simulink model "NOx_INTEGRATED_GUIDLINE_MODEL"  (R2019a)
settings: Solver=FixedStepDiscrete  StartTime=0.0  StopTime=100  FixedStep=0.1  RelTol=1e-3
values from neighbouring files (symbols this model uses):
  ADblue_CONC_MAX = 34.0    [Integrated_Model_DD.sldd]    (also in NOx_INTEGRATED_PARAMETER_SCRIPT.m = Simulink.Parameter)
  ADblue_CONC_MIN = 33.0    [Integrated_Model_DD.sldd]    (also in NOx_INTEGRATED_PARAMETER_SCRIPT.m = Simulink.Parameter)
  ADblue_LEVEL_MAX = 30.0    [Integrated_Model_DD.sldd]    (also in NOx_INTEGRATED_PARAMETER_SCRIPT.m = Simulink.Parameter)
  ADblue_LEVEL_MIN = 15.0    [Integrated_Model_DD.sldd]    (also in NOx_INTEGRATED_PARAMETER_SCRIPT.m = Simulink.Parameter)
  FLOW_RATE_MIN = 4.8    [Integrated_Model_DD.sldd]    (also in NOx_INTEGRATED_PARAMETER_SCRIPT.m = Simulink.Parameter)
  HEATER = 5.0    [Integrated_Model_DD.sldd]    (also in NOx_INTEGRATED_PARAMETER_SCRIPT.m = Simulink.Parameter)
  NOX_DOWN = 10.0    [Integrated_Model_DD.sldd]    (also in NOx_INTEGRATED_PARAMETER_SCRIPT.m = Simulink.Parameter)
  O2_concentration_max = 14.0    [Integrated_Model_DD.sldd]    (also in NOx_INTEGRATED_PARAMETER_SCRIPT.m = Simulink.Parameter)
  O2_concentration_min = 8.0    [Integrated_Model_DD.sldd]    (also in NOx_INTEGRATED_PARAMETER_SCRIPT.m = Simulink.Parameter)
  PRESSURE_REQ = 5.8    [Integrated_Model_DD.sldd]    (also in NOx_INTEGRATED_PARAMETER_SCRIPT.m = Simulink.Parameter)
  REG_TIME_OFF = 25.0    [Integrated_Model_DD.sldd]    (also in NOx_INTEGRATED_PARAMETER_SCRIPT.m = Simulink.Parameter)
  SCR_BED_TEMP_MIN = 200.0    [Integrated_Model_DD.sldd]    (also in NOx_INTEGRATED_PARAMETER_SCRIPT.m = Simulink.Parameter)
  soot_max = 0.45    [Integrated_Model_DD.sldd]    (also in NOx_INTEGRATED_PARAMETER_SCRIPT.m = Simulink.Parameter)
  soot_mil = 0.9    [Integrated_Model_DD.sldd]    (also in NOx_INTEGRATED_PARAMETER_SCRIPT.m = Simulink.Parameter)
  Time_off = 0.0    [Integrated_Model_DD.sldd]    (also in NOx_INTEGRATED_PARAMETER_SCRIPT.m = Simulink.Parameter)
  Time_on = 1.0    [Integrated_Model_DD.sldd]    (also in NOx_INTEGRATED_PARAMETER_SCRIPT.m = Simulink.Parameter)
  TIMER = 0.1    [Integrated_Model_DD.sldd]    (also in NOx_INTEGRATED_PARAMETER_SCRIPT.m = Simulink.Parameter)
settings Model: Creator=User  LastModifiedBy=User
settings OptimizationCC: DefaultParameterBehavior=Inlined  EnhancedBackFolding=on  PassReuseOutputArgsAs=Individual arguments  OptimizeBlockOrder=speed  DifferentSizesBufferReuse=on  OptimizationCustomize=off
settings DebuggingCC: SignalInfNanChecking=warning  ParameterTunabilityLossMsg=error  UniqueDataStoreMsg=warning  StrictBusMsg=ErrorOnBusTreatedAsVector
settings SFSimCC: MATLABDynamicMemAlloc=off
settings RTWCC: SystemTargetFile=ert.tlc  GenCodeOnly=on  TemplateMakefile=ert_default_tmf  GenerateReport=on  IncludeHyperlinkInReport=on  LaunchReport=on  GenerateTraceInfo=on  GenerateTraceReport=on  GenerateTraceReportSl=on  GenerateTraceReportSf=on  GenerateTraceReportEml=on
settings CodeAppCC: ForceParamTrailComments=on  IgnoreCustomStorageClasses=off  OperatorAnnotations=on  SimulinkDataObjDesc=on  SFDataObjDesc=on  InsertBlockDesc=on
settings ERTTargetCC: TargetLangStandard=C99 (ISO)  GenerateSampleERTMain=on  InlinedParameterPlacement=NonHierarchical  ERTCustomFileTemplate=example_file_process.tlc

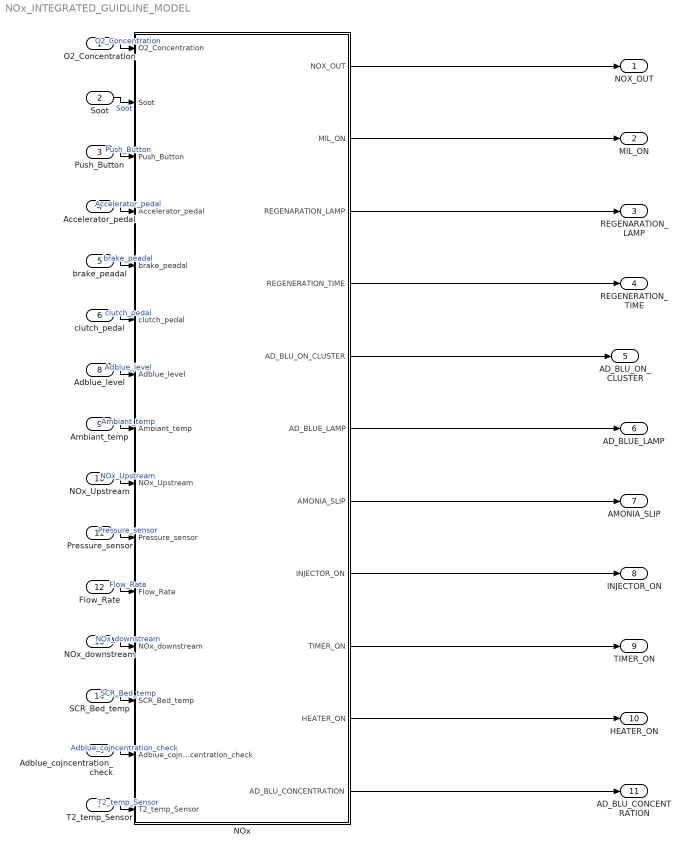
== system NOx_INTEGRATED_GUIDLINE_MODEL ==
  O2_Concentration : Inport
  Soot : Inport  Port=2
  Push_Button : Inport  Port=3
  Accelerator_pedal : Inport  Port=4
  brake_peadal : Inport  Port=5
  clutch_pedal : Inport  Port=6
  T2_temp_Sensor : Inport  Port=7
  Adblue_level : Inport  Port=8
  Ambiant_temp : Inport  Port=9
  NOx_Upstream : Inport  Port=10
  Pressure_sensor : Inport  Port=11
  Flow_Rate : Inport  Port=12
  NOx_downstream : Inport  Port=13
  SCR_Bed_temp : Inport  Port=14
  Adblue_cojncentration_check : Inport  Port=15
  NOx : Subsystem  TreatAsAtomicUnit=on
  NOX_OUT : Outport
  MIL_ON : Outport  Port=2
  REGENARATION_LAMP : Outport  Port=3
  REGENERATION_TIME : Outport  Port=4
  AD_BLU_ON_CLUSTER : Outport  Port=5
  AD_BLUE_LAMP : Outport  Port=6
  AMONIA_SLIP : Outport  Port=7
  INJECTOR_ON : Outport  Port=8
  TIMER_ON : Outport  Port=9
  HEATER_ON : Outport  Port=10
  AD_BLU_CONCENTRATION : Outport  Port=11
  wires:
  Adblue_cojncentration_check/1 -> NOx/14(Adblue_cojncentration_check)  "Adblue_cojncentration_check"
  Pressure_sensor/1 -> NOx/10(Pressure_sensor)  "Pressure_sensor"
  Flow_Rate/1 -> NOx/11(Flow_Rate)  "Flow_Rate"
  T2_temp_Sensor/1 -> NOx/15(T2_temp_Sensor)  "T2_temp_Sensor"
  SCR_Bed_temp/1 -> NOx/13(SCR_Bed_temp)  "SCR_Bed_temp"
  Soot/1 -> NOx/2(Soot)  "Soot"
  NOx_downstream/1 -> NOx/12(NOx_downstream)  "NOx_downstream"
  NOx_Upstream/1 -> NOx/9(NOx_Upstream)  "NOx_Upstream"
  O2_Concentration/1 -> NOx/1(O2_Concentration)  "O2_Concentration"
  Ambiant_temp/1 -> NOx/8(Ambiant_temp)  "Ambiant_temp"
  brake_peadal/1 -> NOx/5(brake_peadal)  "brake_peadal"
  Accelerator_pedal/1 -> NOx/4(Accelerator_pedal)  "Accelerator_pedal"
  Push_Button/1 -> NOx/3(Push_Button)  "Push_Button"
  clutch_pedal/1 -> NOx/6(clutch_pedal)  "clutch_pedal"
  Adblue_level/1 -> NOx/7(Adblue_level)  "Adblue_level"
  NOx/2(MIL_ON) -> MIL_ON/1
  NOx/11(AD_BLU_CONCENTRATION) -> AD_BLU_CONCENTRATION/1
  NOx/6(AD_BLUE_LAMP) -> AD_BLUE_LAMP/1
  NOx/1(NOX_OUT) -> NOX_OUT/1
  NOx/7(AMONIA_SLIP) -> AMONIA_SLIP/1
  NOx/4(REGENERATION_TIME) -> REGENERATION_TIME/1
  NOx/3(REGENARATION_LAMP) -> REGENARATION_LAMP/1
  NOx/8(INJECTOR_ON) -> INJECTOR_ON/1
  NOx/5(AD_BLU_ON_CLUSTER) -> AD_BLU_ON_CLUSTER/1
  NOx/10(HEATER_ON) -> HEATER_ON/1
  NOx/9(TIMER_ON) -> TIMER_ON/1

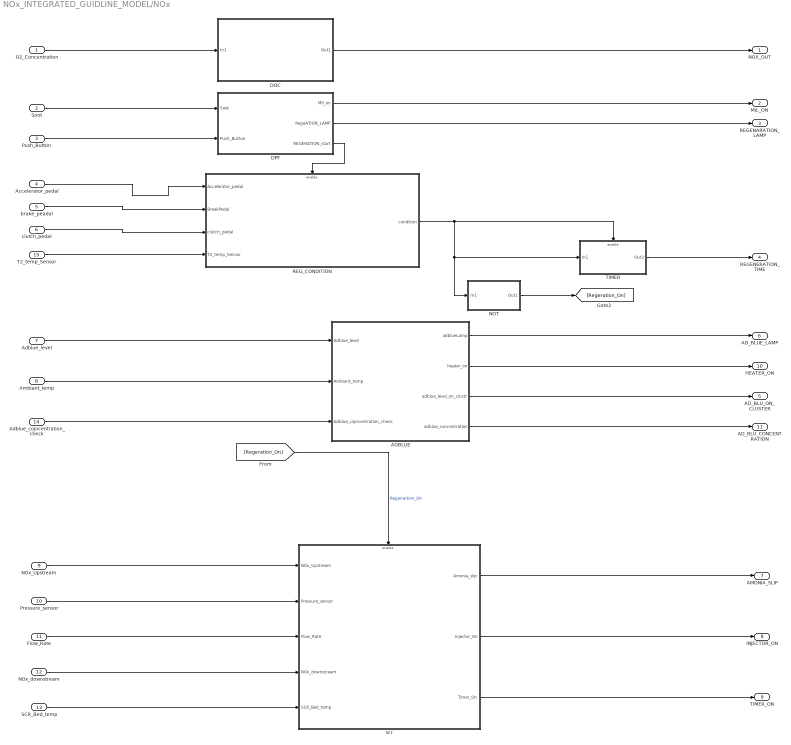
== system NOx_INTEGRATED_GUIDLINE_MODEL/NOx ==
  O2_Concentration : Inport
  Soot : Inport  Port=2
  Push_Button : Inport  Port=3
  Accelerator_pedal : Inport  Port=4
  brake_peadal : Inport  Port=5
  clutch_pedal : Inport  Port=6
  Adblue_level : Inport  Port=7
  Ambiant_temp : Inport  Port=8
  NOx_Upstream : Inport  Port=9
  Pressure_sensor : Inport  Port=10
  Flow_Rate : Inport  Port=11
  NOx_downstream : Inport  Port=12
  SCR_Bed_temp : Inport  Port=13
  Adblue_cojncentration_check : Inport  Port=14
  T2_temp_Sensor : Inport  Port=15
  ADBLUE : Subsystem  TreatAsAtomicUnit=on
  DOC : Subsystem  TreatAsAtomicUnit=on
  DPF : Subsystem  TreatAsAtomicUnit=on
  NOT : Subsystem  TreatAsAtomicUnit=on
  REG_CONDITION : Subsystem
  TIMER : Subsystem
  scr : Subsystem
  NOX_OUT : Outport
  MIL_ON : Outport  Port=2
  REGENARATION_LAMP : Outport  Port=3
  REGENERATION_TIME : Outport  Port=4
  AD_BLU_ON_CLUSTER : Outport  Port=5
  AD_BLUE_LAMP : Outport  Port=6
  AMONIA_SLIP : Outport  Port=7
  INJECTOR_ON : Outport  Port=8
  TIMER_ON : Outport  Port=9
  HEATER_ON : Outport  Port=10
  AD_BLU_CONCENTRATION : Outport  Port=11
  wires:
  scr/3(Timer_On) -> TIMER_ON/1
  Push_Button/1 -> DPF/2(Push_Button)
  DPF/3(REGERATION_start) -> REG_CONDITION/Enable
  scr/1(Amonia_slip) -> AMONIA_SLIP/1
  NOx_Upstream/1 -> scr/1(NOx_Upstream)
  DOC/1(Out1) -> NOX_OUT/1
  DPF/2(RegeATION_LAMP) -> REGENARATION_LAMP/1
  [Regeration_On] -> scr/Enable  "Regenartion_On"
  Adblue_level/1 -> ADBLUE/1(Adblue_level)
  O2_Concentration/1 -> DOC/1(In1)
  Accelerator_pedal/1 -> REG_CONDITION/1(Accelerator_pedal)
  Flow_Rate/1 -> scr/3(Flow_Rate)
  Soot/1 -> DPF/1(Soot)
  Pressure_sensor/1 -> scr/2(Pressure_sensor)
  scr/2(Injector_On) -> INJECTOR_ON/1
  NOx_downstream/1 -> scr/4(NOx_downstream)
  SCR_Bed_temp/1 -> scr/5(SCR_Bed_temp)
  DPF/1(MIl_on) -> MIL_ON/1
  Ambiant_temp/1 -> ADBLUE/2(Ambiant_temp)
  ADBLUE/1(adblueLamp) -> AD_BLUE_LAMP/1
  ADBLUE/3(adblue_level_on_clustr) -> AD_BLU_ON_CLUSTER/1
  ADBLUE/2(heater_on) -> HEATER_ON/1
  Adblue_cojncentration_check/1 -> ADBLUE/3(Adblue_cojncentration_check)
  ADBLUE/4(adblue_concentration) -> AD_BLU_CONCENTRATION/1
  TIMER/1(Out2) -> REGENERATION_TIME/1
  clutch_pedal/1 -> REG_CONDITION/3(clutch_pedal)
  brake_peadal/1 -> REG_CONDITION/2(BreakPedal)
  T2_temp_Sensor/1 -> REG_CONDITION/4(T2_temp_Sensor)
  NOT/1(Out1) -> [Regeration_On]
  REG_CONDITION/1(condition) -> TIMER/1(In1), NOT/1(In1), TIMER/Enable

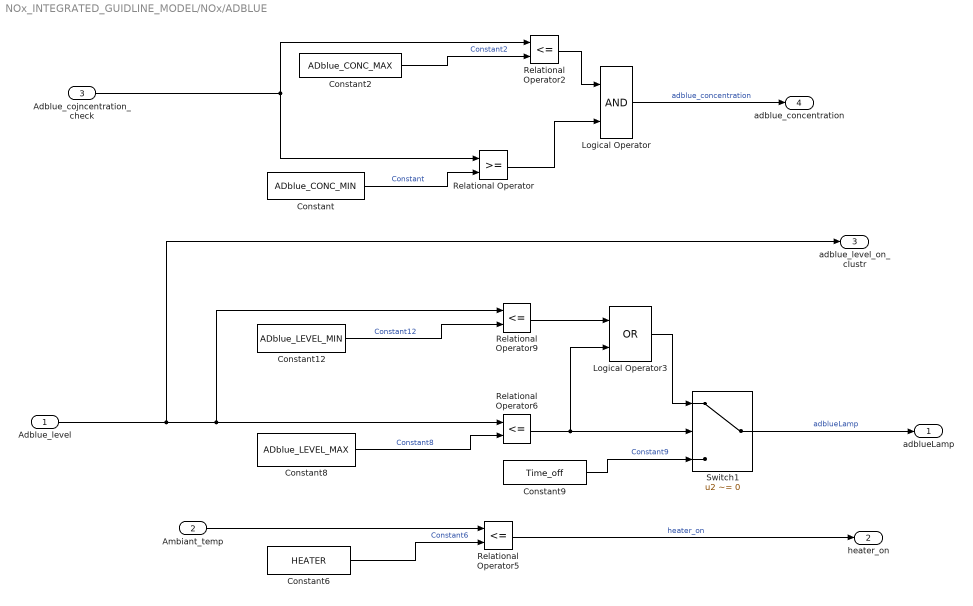
== system NOx_INTEGRATED_GUIDLINE_MODEL/NOx/ADBLUE ==
  Adblue_level : Inport
  Ambiant_temp : Inport  Port=2
  Adblue_cojncentration_check : Inport  Port=3
  Constant : Constant  Value=ADblue_CONC_MIN
  Constant12 : Constant  Value=ADblue_LEVEL_MIN
  Constant2 : Constant  Value=ADblue_CONC_MAX
  Constant6 : Constant  Value=HEATER  OutDataTypeStr=int8
  Constant8 : Constant  Value=ADblue_LEVEL_MAX
  Constant9 : Constant  Value=Time_off
  Logical Operator : Logic  AllPortsSameDT=off  OutDataTypeStr=boolean
  Logical Operator3 : Logic  Operator=OR  AllPortsSameDT=off  OutDataTypeStr=boolean
  Relational Operator : RelationalOperator  OutDataTypeStr=boolean  RndMeth=Simplest
  Relational Operator{2,5..6,9} (4 alike) : RelationalOperator  Operator=<=  OutDataTypeStr=boolean  RndMeth=Simplest
  Switch1 : Switch  Criteria=u2 ~= 0
  adblueLamp : Outport
  heater_on : Outport  Port=2
  adblue_level_on_clustr : Outport  Port=3
  adblue_concentration : Outport  Port=4
  wires:
  Logical Operator3/1 -> Switch1/1
  Constant9/1 -> Switch1/3  "Constant9"
  Adblue_level/1 -> adblue_level_on_clustr/1, Relational Operator6/1, Relational Operator9/1
  Constant8/1 -> Relational Operator6/2  "Constant8"
  Constant12/1 -> Relational Operator9/2  "Constant12"
  Relational Operator6/1 -> Logical Operator3/2, Switch1/2
  Constant6/1 -> Relational Operator5/2  "Constant6"
  Relational Operator5/1 -> heater_on/1  "heater_on"
  Switch1/1 -> adblueLamp/1  "adblueLamp"
  Ambiant_temp/1 -> Relational Operator5/1
  Constant/1 -> Relational Operator/2  "Constant"
  Constant2/1 -> Relational Operator2/2  "Constant2"
  Relational Operator2/1 -> Logical Operator/1
  Adblue_cojncentration_check/1 -> Relational Operator/1, Relational Operator2/1
  Logical Operator/1 -> adblue_concentration/1  "adblue_concentration"
  Relational Operator/1 -> Logical Operator/2
  Relational Operator9/1 -> Logical Operator3/1

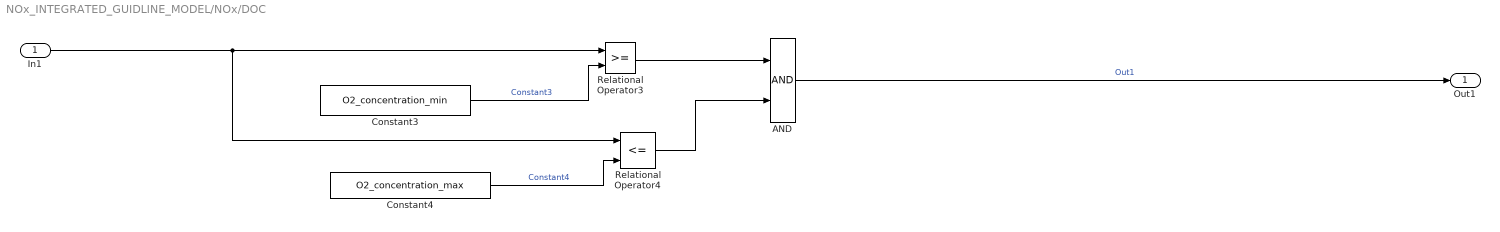
== system NOx_INTEGRATED_GUIDLINE_MODEL/NOx/DOC ==
  In1 : Inport
  AND : Logic  AllPortsSameDT=off  OutDataTypeStr=boolean
  Constant3 : Constant  Value=O2_concentration_min
  Constant4 : Constant  Value=O2_concentration_max
  Relational Operator3 : RelationalOperator  OutDataTypeStr=boolean  RndMeth=Simplest
  Relational Operator4 : RelationalOperator  Operator=<=  OutDataTypeStr=boolean  RndMeth=Simplest
  Out1 : Outport
  wires:
  Constant3/1 -> Relational Operator3/2  "Constant3"
  Relational Operator3/1 -> AND/1
  AND/1 -> Out1/1  "Out1"
  In1/1 -> Relational Operator4/1, Relational Operator3/1
  Constant4/1 -> Relational Operator4/2  "Constant4"
  Relational Operator4/1 -> AND/2

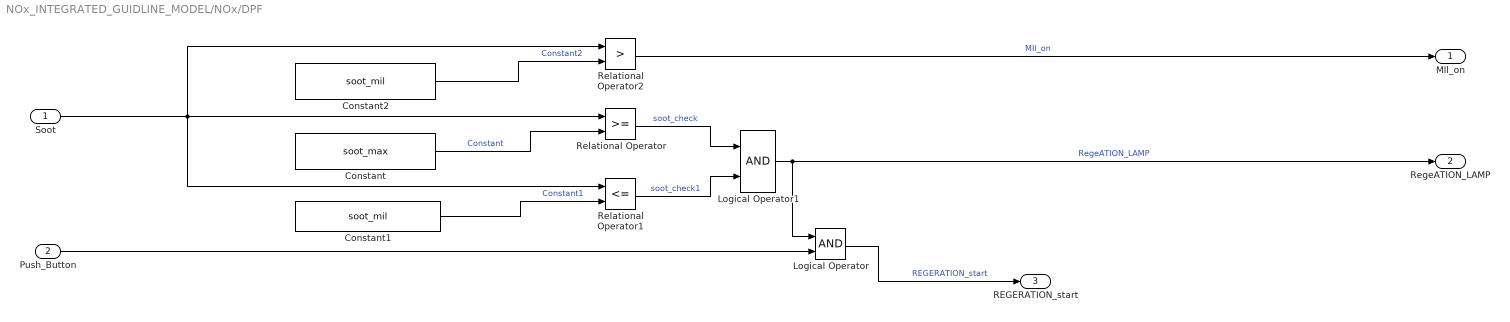
== system NOx_INTEGRATED_GUIDLINE_MODEL/NOx/DPF ==
  Soot : Inport
  Push_Button : Inport  Port=2
  Constant : Constant  Value=soot_max
  Constant1 : Constant  Value=soot_mil
  Constant2 : Constant  Value=soot_mil
  Logical Operator : Logic  AllPortsSameDT=off  OutDataTypeStr=boolean
  Logical Operator1 : Logic  AllPortsSameDT=off  OutDataTypeStr=boolean
  Relational Operator : RelationalOperator  OutDataTypeStr=boolean  RndMeth=Simplest
  Relational Operator1 : RelationalOperator  Operator=<=  OutDataTypeStr=boolean  RndMeth=Simplest
  Relational Operator2 : RelationalOperator  Operator=>  OutDataTypeStr=boolean  RndMeth=Simplest
  MIl_on : Outport
  RegeATION_LAMP : Outport  Port=2
  REGERATION_start : Outport  Port=3
  wires:
  Soot/1 -> Relational Operator1/1, Relational Operator2/1, Relational Operator/1
  Logical Operator/1 -> REGERATION_start/1  "REGERATION_start"
  Logical Operator1/1 -> RegeATION_LAMP/1, Logical Operator/1  "RegeATION_LAMP"
  Constant2/1 -> Relational Operator2/2  "Constant2"
  Push_Button/1 -> Logical Operator/2
  Constant1/1 -> Relational Operator1/2  "Constant1"
  Constant/1 -> Relational Operator/2  "Constant"
  Relational Operator1/1 -> Logical Operator1/2  "soot_check1"
  Relational Operator2/1 -> MIl_on/1  "MIl_on"
  Relational Operator/1 -> Logical Operator1/1  "soot_check"

== system NOx_INTEGRATED_GUIDLINE_MODEL/NOx/NOT ==
  In1 : Inport
  NOT : Logic  Operator=NOT  IconShape=distinctive  AllPortsSameDT=off  OutDataTypeStr=boolean
  Out1 : Outport
  wires:
  In1/1 -> NOT/1
  NOT/1 -> Out1/1  "not_out"

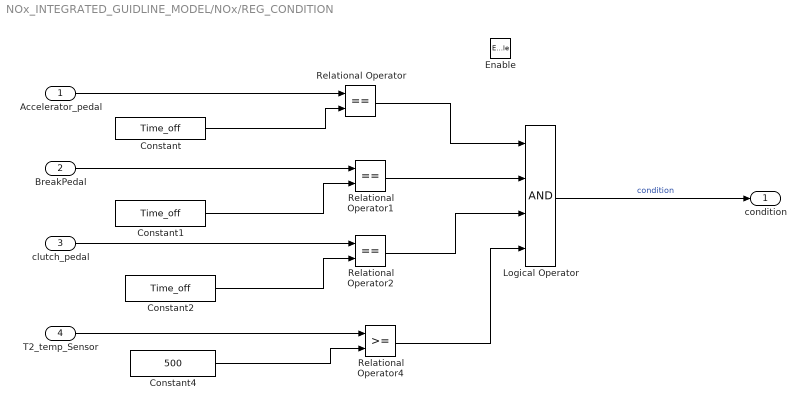
== system NOx_INTEGRATED_GUIDLINE_MODEL/NOx/REG_CONDITION ==
  Accelerator_pedal : Inport
  BreakPedal : Inport  Port=2
  clutch_pedal : Inport  Port=3
  T2_temp_Sensor : Inport  Port=4
  Enable : EnablePort  StatesWhenEnabling=reset
  Constant : Constant  Value=Time_off
  Constant1 : Constant  Value=Time_off
  Constant2 : Constant  Value=Time_off
  Constant4 : Constant  Value=500
  Logical Operator : Logic  Inputs=4  AllPortsSameDT=off
  Relational Operator : RelationalOperator  Operator===  OutDataTypeStr=boolean  RndMeth=Simplest
  Relational Operator1 : RelationalOperator  Operator===  OutDataTypeStr=boolean  RndMeth=Simplest
  Relational Operator2 : RelationalOperator  Operator===  OutDataTypeStr=boolean  RndMeth=Simplest
  Relational Operator4 : RelationalOperator  OutDataTypeStr=boolean  RndMeth=Simplest
  condition : Outport
  wires:
  Constant/1 -> Relational Operator/2
  Accelerator_pedal/1 -> Relational Operator/1
  Constant1/1 -> Relational Operator1/2
  Constant2/1 -> Relational Operator2/2
  Relational Operator/1 -> Logical Operator/1
  Relational Operator1/1 -> Logical Operator/2
  Relational Operator2/1 -> Logical Operator/3
  Constant4/1 -> Relational Operator4/2
  Logical Operator/1 -> condition/1  "condition"
  Relational Operator4/1 -> Logical Operator/4
  BreakPedal/1 -> Relational Operator1/1
  clutch_pedal/1 -> Relational Operator2/1
  T2_temp_Sensor/1 -> Relational Operator4/1

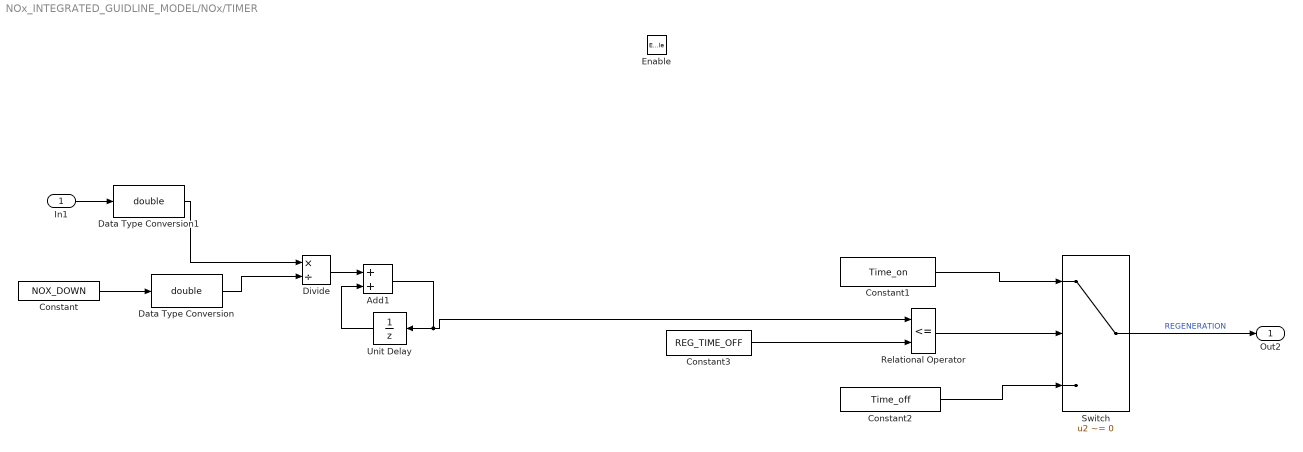
== system NOx_INTEGRATED_GUIDLINE_MODEL/NOx/TIMER ==
  In1 : Inport
  Enable : EnablePort  StatesWhenEnabling=reset
  Add1 : Sum  OutDataTypeStr=double
  Constant : Constant  Value=NOX_DOWN  OutDataTypeStr=double
  Constant1 : Constant  Value=Time_on
  Constant2 : Constant  Value=Time_off
  Constant3 : Constant  Value=REG_TIME_OFF
  Data Type Conversion : DataTypeConversion  OutDataTypeStr=double
  Data Type Conversion1 : DataTypeConversion  OutDataTypeStr=double
  Divide : Product  Inputs=*/  OutDataTypeStr=double
  Relational Operator : RelationalOperator  Operator=<=  OutDataTypeStr=boolean  RndMeth=Simplest
  Switch : Switch  Criteria=u2 ~= 0
  Unit Delay : UnitDelay  InitialCondition=0.1  SampleTime=-1  HasFrameUpgradeWarning=on
  Out2 : Outport
  wires:
  Unit Delay/1 -> Add1/2
  Divide/1 -> Add1/1
  Constant/1 -> Data Type Conversion/1
  Add1/1 -> Relational Operator/1, Unit Delay/1
  Constant2/1 -> Switch/3
  Constant3/1 -> Relational Operator/2
  Switch/1 -> Out2/1  "REGENERATION"
  Relational Operator/1 -> Switch/2
  Constant1/1 -> Switch/1
  In1/1 -> Data Type Conversion1/1
  Data Type Conversion/1 -> Divide/2
  Data Type Conversion1/1 -> Divide/1

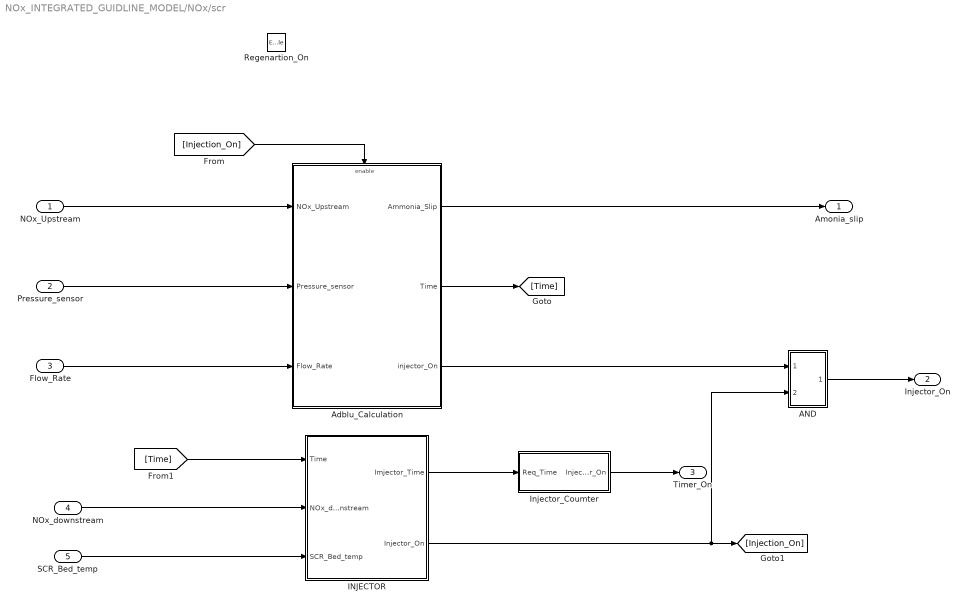
== system NOx_INTEGRATED_GUIDLINE_MODEL/NOx/scr ==
  NOx_Upstream : Inport
  Pressure_sensor : Inport  Port=2
  Flow_Rate : Inport  Port=3
  NOx_downstream : Inport  Port=4
  SCR_Bed_temp : Inport  Port=5
  Regenartion_On : EnablePort
  AND : Subsystem  TreatAsAtomicUnit=on
  Adblu_Calculation : Subsystem
  INJECTOR : Subsystem
  Injector_Coumter : Subsystem  TreatAsAtomicUnit=on
  Amonia_slip : Outport
  Injector_On : Outport  Port=2
  Timer_On : Outport  Port=3
  wires:
  Adblu_Calculation/2(Time) -> [Time]
  [Time] -> INJECTOR/1(Time)
  Injector_Coumter/1(Injector_On) -> Timer_On/1
  INJECTOR/2(Injector_On) -> [Injection_On], AND/2(In2)
  INJECTOR/1(Imjector_Time) -> Injector_Coumter/1(Req_Time)
  [Injection_On] -> Adblu_Calculation/Enable
  Adblu_Calculation/1(Ammonia_Slip) -> Amonia_slip/1
  NOx_downstream/1 -> INJECTOR/2(NOx_downstream)
  NOx_Upstream/1 -> Adblu_Calculation/1(NOx_Upstream)
  SCR_Bed_temp/1 -> INJECTOR/3(SCR_Bed_temp)
  Pressure_sensor/1 -> Adblu_Calculation/2(Pressure_sensor)
  Flow_Rate/1 -> Adblu_Calculation/3(Flow_Rate)
  Adblu_Calculation/3(injector_On) -> AND/1(In1)
  AND/1(Out1) -> Injector_On/1

== system NOx_INTEGRATED_GUIDLINE_MODEL/NOx/scr/AND ==
  In1 : Inport
  In2 : Inport  Port=2
  Logical Operator2 : Logic  AllPortsSameDT=off  OutDataTypeStr=boolean
  Out1 : Outport
  wires:
  In2/1 -> Logical Operator2/2
  Logical Operator2/1 -> Out1/1  "Out1"
  In1/1 -> Logical Operator2/1

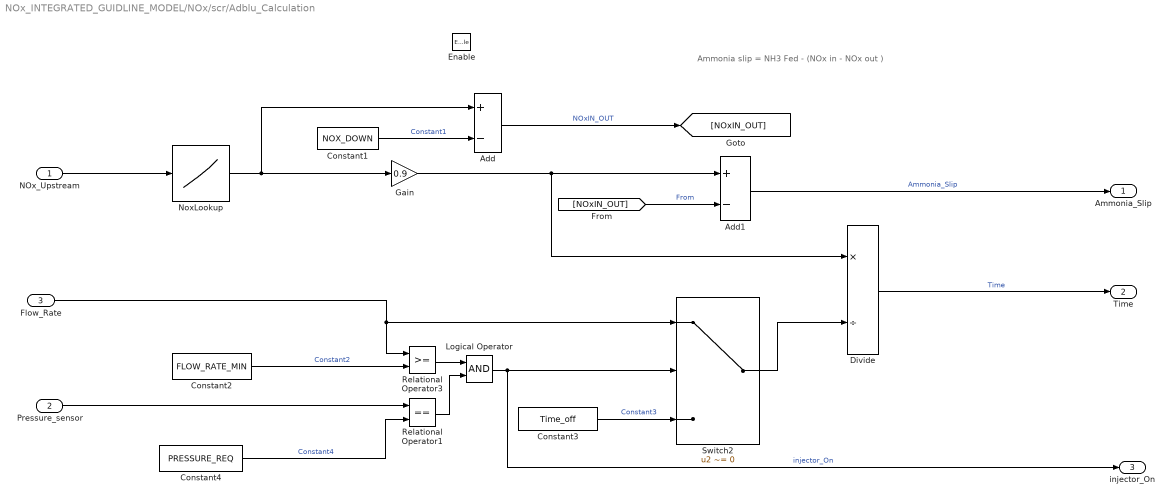
== system NOx_INTEGRATED_GUIDLINE_MODEL/NOx/scr/Adblu_Calculation ==
  note: Ammonia slip = NH3 Fed - (NOx in - NOx out )
  NOx_Upstream : Inport
  Pressure_sensor : Inport  Port=2
  Flow_Rate : Inport  Port=3
  Enable : EnablePort  StatesWhenEnabling=reset
  Add : Sum  Inputs=+-
  Add1 : Sum  Inputs=+-
  Constant1 : Constant  Value=NOX_DOWN
  Constant2 : Constant  Value=FLOW_RATE_MIN
  Constant3 : Constant  Value=Time_off
  Constant4 : Constant  Value=PRESSURE_REQ
  Divide : Product  Inputs=*/  OutDataTypeStr=double  RndMeth=Round
  Gain : Gain  Gain=0.9
  Logical Operator : Logic  AllPortsSameDT=off  OutDataTypeStr=boolean
  NoxLookup : Lookup_n-D  NumberOfTableDimensions=1  BreakpointsForDimension1=|  BreakpointsForDimension1DataTypeStr=double  Table=|  TableDataTypeStr=double  IntermediateResultsDataTypeStr=double  InternalRulePriority=Speed  OutDataTypeStr=double  InputSameDT=on
      BreakpointsForDimension1=|
      | [10
      | 70
      | 77.6
      | 80.4
      | 86.4
      | 99.6
      | 108
      | 117.6
      | 127.2
      | 136.8
      | 149.3
      | 158.3
      | 163.3
      | 168.3
      | 175.3
      | 181.5
      | 187.7
      | 193.9
      | 200.1
      | 206.3
      | 212.85
      | 223.5
      | 233.15
      | 242.8
      | 255.45
      | 264.9
      | 275.35
      | 285.8
      | 296.25
      | 306.7
      | 317.15
      | 327.6
      | 338.05
      | 348.5
      | 358.95
      | 369.4
      | 379.85
      | 390.3
      | 400.75
      | 411.2
      | 421.65
      | 432.1
      | 442.55
      | 453
      | 463.45
      | 473.9
      | 484.35
      | 494.8
      | 505.25
      | 515.7
      | 526.15
      | 536.6
      | 547.05
      | 557.5
      | 567.95
      | 578.4
      | 588.85
      | 599.3
      | 609.75
      | 620.2
      | 630.65
      | 641.1
      | 651.55
      | 662
      | 672.45
      | 682.9
      | 693.35
      | 703.8
      | ]
      Table=|
      | [10
      | 70
      | 77.6
      | 80.4
      | 86.4
      | 99.6
      | 108
      | 117.6
      | 127.2
      | 136.8
      | 149.3
      | 158.3
      | 163.3
      | 168.3
      | 175.3
      | 181.5
      | 187.7
      | 193.9
      | 200.1
      | 206.3
      | 212.85
      | 223.5
      | 233.15
      | 242.8
      | 255.45
      | 264.9
      | 275.35
      | 285.8
      | 296.25
      | 306.7
      | 317.15
      | 327.6
      | 338.05
      | 348.5
      | 358.95
      | 369.4
      | 379.85
      | 390.3
      | 400.75
      | 411.2
      | 421.65
      | 432.1
      | 442.55
      | 453
      | 463.45
      | 473.9
      | 484.35
      | 494.8
      | 505.25
      | 515.7
      | 526.15
      | 536.6
      | 547.05
      | 557.5
      | 567.95
      | 578.4
      | 588.85
      | 599.3
      | 609.75
      | 620.2
      | 630.65
      | 641.1
      | 651.55
      | 662
      | 672.45
      | 682.9
      | 693.35
      | 703.8
      | ]
  Relational Operator1 : RelationalOperator  Operator===  OutDataTypeStr=boolean  RndMeth=Simplest
  Relational Operator3 : RelationalOperator  OutDataTypeStr=boolean  RndMeth=Simplest
  Switch2 : Switch  Criteria=u2 ~= 0
  Ammonia_Slip : Outport
  Time : Outport  Port=2
  injector_On : Outport  Port=3
  wires:
  Pressure_sensor/1 -> Relational Operator1/1
  Add/1 -> [NOxIN_OUT]  "NOxIN_OUT"
  Constant1/1 -> Add/2  "Constant1"
  Relational Operator1/1 -> Logical Operator/2
  Constant4/1 -> Relational Operator1/2  "Constant4"
  NOx_Upstream/1 -> NoxLookup/1
  Constant2/1 -> Relational Operator3/2  "Constant2"
  Relational Operator3/1 -> Logical Operator/1
  Constant3/1 -> Switch2/3  "Constant3"
  Switch2/1 -> Divide/2
  Logical Operator/1 -> injector_On/1, Switch2/2  "injector_On"
  [NOxIN_OUT] -> Add1/2  "From"
  Flow_Rate/1 -> Relational Operator3/1, Switch2/1
  Add1/1 -> Ammonia_Slip/1  "Ammonia_Slip"
  Gain/1 -> Divide/1, Add1/1
  Divide/1 -> Time/1  "Time"
  NoxLookup/1 -> Gain/1, Add/1

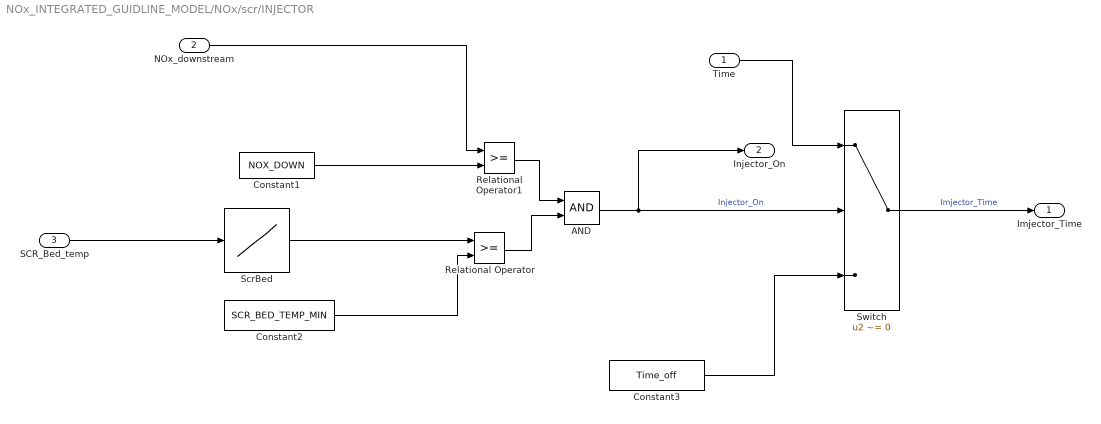
== system NOx_INTEGRATED_GUIDLINE_MODEL/NOx/scr/INJECTOR ==
  Time : Inport
  NOx_downstream : Inport  Port=2
  SCR_Bed_temp : Inport  Port=3
  AND : Logic  AllPortsSameDT=off  OutDataTypeStr=boolean
  Constant1 : Constant  Value=NOX_DOWN
  Constant2 : Constant  Value=SCR_BED_TEMP_MIN
  Constant3 : Constant  Value=Time_off
  Relational Operator : RelationalOperator  OutDataTypeStr=boolean  RndMeth=Simplest
  Relational Operator1 : RelationalOperator  OutDataTypeStr=boolean  RndMeth=Simplest
  ScrBed : Lookup_n-D  NumberOfTableDimensions=1  BreakpointsForDimension1=[1:10:650]  BreakpointsForDimension2=[1:1:500]  BreakpointsForDimension1DataTypeStr=double  Table=[1:10:650]  TableDataTypeStr=double  IntermediateResultsDataTypeStr=double  InternalRulePriority=Speed  OutDataTypeStr=double  InputSameDT=on
  Switch : Switch  Criteria=u2 ~= 0
  Imjector_Time : Outport
  Injector_On : Outport  Port=2
  wires:
  Constant1/1 -> Relational Operator1/2
  Constant2/1 -> Relational Operator/2
  Constant3/1 -> Switch/3
  ScrBed/1 -> Relational Operator/1
  AND/1 -> Injector_On/1, Switch/2  "Injector_On"
  Time/1 -> Switch/1
  Relational Operator1/1 -> AND/1
  Relational Operator/1 -> AND/2
  SCR_Bed_temp/1 -> ScrBed/1
  Switch/1 -> Imjector_Time/1  "Imjector_Time"
  NOx_downstream/1 -> Relational Operator1/1

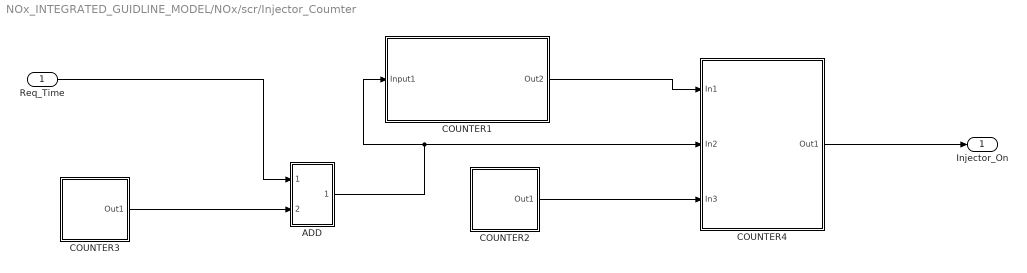
== system NOx_INTEGRATED_GUIDLINE_MODEL/NOx/scr/Injector_Coumter ==
  Req_Time : Inport
  ADD : Subsystem
  COUNTER1 : Subsystem
  COUNTER2 : Subsystem
  COUNTER3 : Subsystem
  COUNTER4 : Subsystem
  Injector_On : Outport
  wires:
  ADD/1(Out1) -> COUNTER4/2(In2), COUNTER1/1(Input1)
  Req_Time/1 -> ADD/1(In1)
  COUNTER1/1(Out2) -> COUNTER4/1(In1)
  COUNTER4/1(Out1) -> Injector_On/1
  COUNTER3/1(Out1) -> ADD/2(In2)
  COUNTER2/1(Out1) -> COUNTER4/3(In3)

== system NOx_INTEGRATED_GUIDLINE_MODEL/NOx/scr/Injector_Coumter/ADD ==
  In1 : Inport
  In2 : Inport  Port=2
  Add1 : Sum
  Relational Operator1 : RelationalOperator  OutDataTypeStr=boolean  RndMeth=Simplest
  Unit Delay : UnitDelay  SampleTime=-1  HasFrameUpgradeWarning=on
  Out1 : Outport
  wires:
  Unit Delay/1 -> Add1/2
  Add1/1 -> Unit Delay/1, Relational Operator1/2
  Relational Operator1/1 -> Out1/1  "Out1"
  In1/1 -> Relational Operator1/1
  In2/1 -> Add1/1

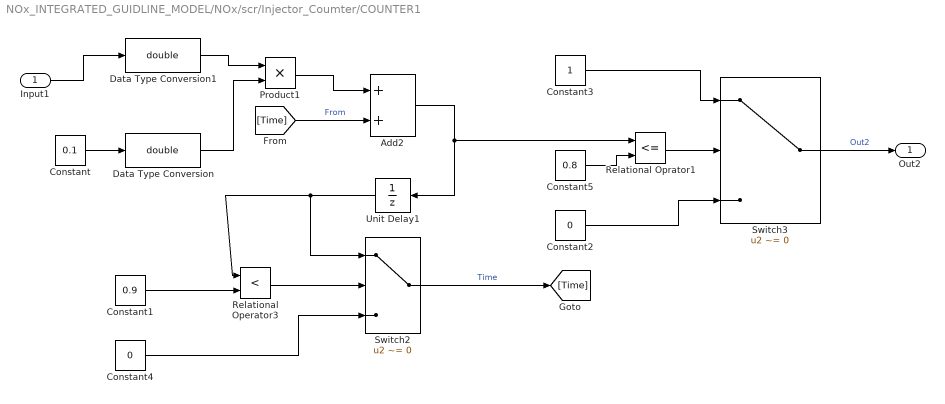
== system NOx_INTEGRATED_GUIDLINE_MODEL/NOx/scr/Injector_Coumter/COUNTER1 ==
  Input1 : Inport
  Add2 : Sum
  Constant : Constant  Value=0.1
  Constant1 : Constant  Value=0.9
  Constant2 : Constant  Value=0
  Constant3 : Constant
  Constant4 : Constant  Value=0
  Constant5 : Constant  Value=0.8
  Data Type Conversion : DataTypeConversion  OutDataTypeStr=double
  Data Type Conversion1 : DataTypeConversion  OutDataTypeStr=double
  Product1 : Product
  Relational Operator3 : RelationalOperator  Operator=<  OutDataTypeStr=boolean  RndMeth=Simplest
  Relational Oprator1 : RelationalOperator  Operator=<=  OutDataTypeStr=boolean  RndMeth=Simplest
  Switch2 : Switch  Criteria=u2 ~= 0
  Switch3 : Switch  Criteria=u2 ~= 0
  Unit Delay1 : UnitDelay  SampleTime=-1  HasFrameUpgradeWarning=on
  Out2 : Outport
  wires:
  Unit Delay1/1 -> Relational Operator3/1, Switch2/1
  Relational Operator3/1 -> Switch2/2
  Constant3/1 -> Switch3/1
  Switch3/1 -> Out2/1  "Out2"
  Constant5/1 -> Relational Oprator1/2
  Constant/1 -> Data Type Conversion/1
  Switch2/1 -> [Time]  "Time"
  Product1/1 -> Add2/1
  Constant1/1 -> Relational Operator3/2
  Constant4/1 -> Switch2/3
  Input1/1 -> Data Type Conversion1/1
  Constant2/1 -> Switch3/3
  [Time] -> Add2/2  "From"
  Relational Oprator1/1 -> Switch3/2
  Add2/1 -> Relational Oprator1/1, Unit Delay1/1
  Data Type Conversion/1 -> Product1/2
  Data Type Conversion1/1 -> Product1/1

== system NOx_INTEGRATED_GUIDLINE_MODEL/NOx/scr/Injector_Coumter/COUNTER2 ==
  Constant1 : Constant  Value=Time_off
  Out1 : Outport
  wires:
  Constant1/1 -> Out1/1  "Out1"

== system NOx_INTEGRATED_GUIDLINE_MODEL/NOx/scr/Injector_Coumter/COUNTER3 ==
  Constant : Constant  Value=TIMER
  Out1 : Outport
  wires:
  Constant/1 -> Out1/1  "Out1"

== system NOx_INTEGRATED_GUIDLINE_MODEL/NOx/scr/Injector_Coumter/COUNTER4 ==
  In1 : Inport
  In2 : Inport  Port=2
  In3 : Inport  Port=3
  Switch : Switch  Criteria=u2 ~= 0
  Out1 : Outport
  wires:
  Switch/1 -> Out1/1  "Out1"
  In1/1 -> Switch/1
  In2/1 -> Switch/2
  In3/1 -> Switch/3
